simulink model "test_co_sim"  (R2020b)
settings: Solver=FixedStepDiscrete  StartTime=0.0  StopTime=10.0  FixedStep=1e-3  RelTol=1e-3
PreLoadFcn:
  | simulink_init
StopFcn:
  | % cleanup
  | if instance.reuse_instance()
  |     instance.error_shutdown("SIMULINK actor did not expect to be reused")
  | end
values from neighbouring files (symbols this model uses):
  Kd_IPF = [0 0 0 0 0 0 0 0 0 0 0 0]    [load_data.m]
  Ki_IPF = [0 0 0 0 0 0 0 0 0 0 0 0]    [load_data.m]
  Kp_IPF = [2 2 2 2 2 2 2 2 2 2 2 2]    [load_data.m]
  Maa = [0.7635    0.2320    0.0658    0.0074    0.0039    0.1363    0.0434    0.0473    0.0270    0.0150    0.0108   -0.0017 ... (first row only)    [load_data.m]
  Ra = [0         0         0         0         0         0         0         0         0         0         0         0 ... (first row only)    [load_data.m]
  T_IPF = diag([1 1 1 1 1 1 1 1 1 1 1 0].')    [load_data.m]
libraries: pid_lib x1
settings Model: Creator=ravenst1  LastModifiedBy=anandh

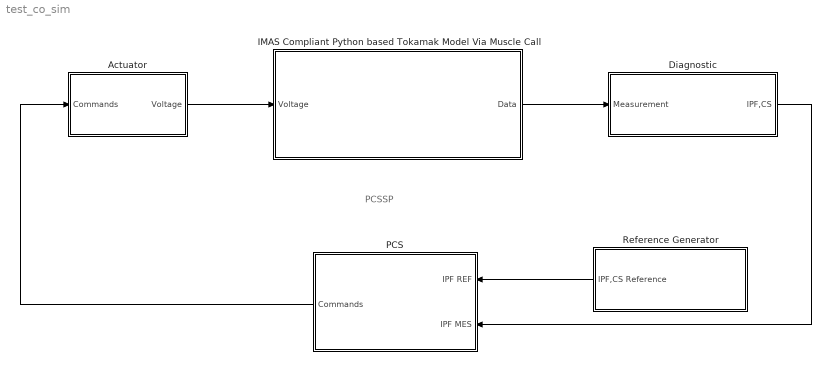
== system test_co_sim ==
  note: PCSSP
  Actuator : Subsystem
  Diagnostic : Subsystem
  "IMAS Compliant Python based Tokamak Model Via Muscle Call " : Subsystem
  PCS : Subsystem
  Reference Generator : Subsystem
  wires:
  PCS/1(Commands) -> Actuator/1(Commands)
  Actuator/1(Voltage) -> "IMAS Compliant Python based Tokamak Model Via Muscle Call "/1(Voltage)
  "IMAS Compliant Python based Tokamak Model Via Muscle Call "/1(Data) -> Diagnostic/1(Measurement)
  Diagnostic/1(IPF,CS) -> PCS/2(IPF MES)
  Reference Generator/1(IPF,CS Reference) -> PCS/1(IPF REF)

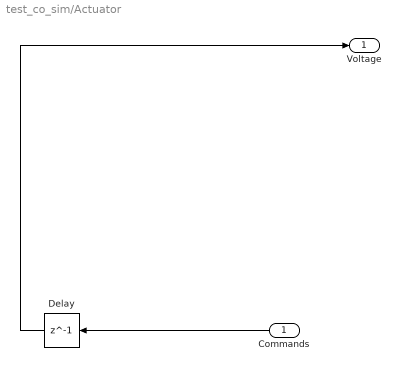
== system test_co_sim/Actuator ==
  Commands : Inport
  Delay : Delay  DelayLength=1
  Voltage : Outport
  wires:
  Commands/1 -> Delay/1
  Delay/1 -> Voltage/1

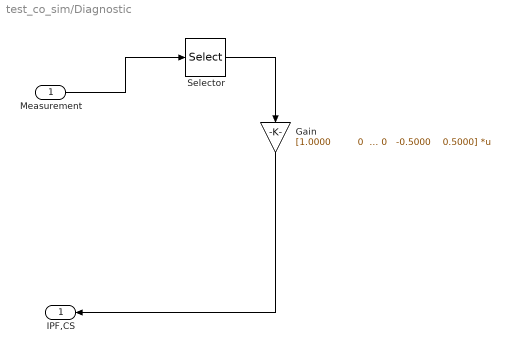
== system test_co_sim/Diagnostic ==
  Measurement : Inport
  Gain : Gain  Gain=|  Multiplication=Matrix(K*u)
      | [1.0000         0         0         0         0         0         0         0         0         0         0         0         0         0
      |          0    1.0000         0         0         0         0         0         0         0         0         0         0         0         0
      |          0         0    0.5000    0.5000         0         0         0         0         0         0         0         0         0         0
      |          0         0         0         0    1.0000         0         0         0         0         0         0         0         0         0
      |          0         0         0         0         0    1.0000         0         0         0         0         0         0         0         0
      |          0         0         0         0         0         0    1.0000         0         0         0         0         0         0         0
      |          0         0         0         0         0         0         0    1.0000         0         0         0         0         0         0
      |          0         0         0         0         0         0         0         0    1.0000         0         0         0         0         0
      |          0         0         0         0         0         0         0         0         0    1.0000         0         0         0         0
      |          0         0         0         0         0         0         0         0         0         0    1.0000         0         0         0
      |          0         0         0         0         0         0         0         0         0         0         0    1.0000         0         0
      |          0         0         0         0         0         0         0         0         0         0         0         0   -0.5000    0.5000]
  Selector : Selector  IndexOptions=Index vector (dialog)  Indices=[iter_system.output_map.cc.start:iter_system.output_map.cc.end]  OutputSizes=1
  IPF,CS : Outport
  wires:
  Selector/1 -> Gain/1
  Measurement/1 -> Selector/1
  Gain/1 -> IPF,CS/1

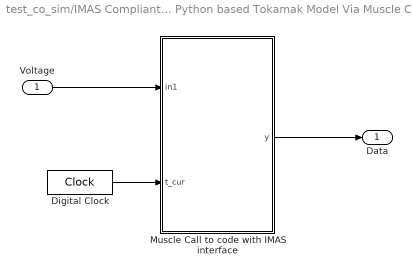
== system test_co_sim/IMAS Compliant Python based Tokamak Model Via Muscle Call  ==
  Voltage : Inport
  Digital Clock : DigitalClock  SampleTime=1e-3
  Muscle Call to code with IMAS interface : MATLAB Function  TreatAsAtomicUnit=on
  Data : Outport
  wires:
  Digital Clock/1 -> Muscle Call to code with IMAS interface/2(t_cur)
  Voltage/1 -> Muscle Call to code with IMAS interface/1(in1)
  Muscle Call to code with IMAS interface/1(y) -> Data/1

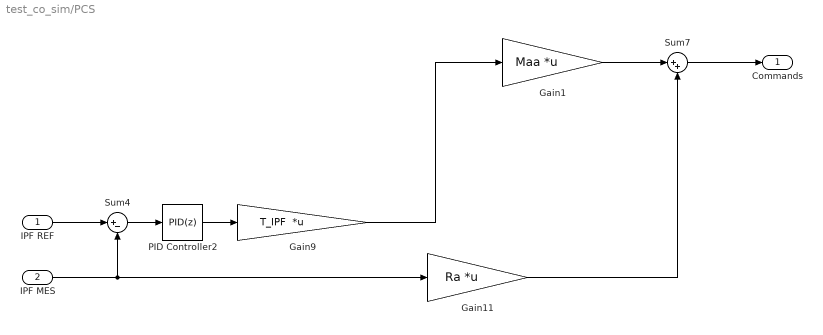
== system test_co_sim/PCS ==
  IPF REF : Inport
  IPF MES : Inport  Port=2
  Gain1 : Gain  Gain=Maa  Multiplication=Matrix(K*u)
  Gain11 : Gain  Gain=Ra  Multiplication=Matrix(K*u)
  Gain9 : Gain  Gain=T_IPF  Multiplication=Matrix(K*u)
  PID Controller2 : pid_lib/PID Controller  Controller=PID  Form=Parallel  TimeDomain=Discrete-time  UseExternalTs=off  SampleTime=-1  IntegratorMethod=Forward Euler  FilterMethod=Forward Euler  ControllerParametersSource=internal  P=Kp_IPF  I=Ki_IPF  D=Kd_IPF  UseFilter=on  N=100  TunerSelectOption=Transfer Function Based (PID Tuner App)  InitialConditionSource=internal  InitialConditionForIntegrator=0  InitialConditionForFilter=0  DifferentiatorICPrevScaledInput=0  ExternalReset=none  TrackingMode=off  Kt=1  LimitOutput=off  SatLimitsSource=internal  UpperSaturationLimit=inf  LowerSaturationLimit=-inf  LinearizeAsGain=on  AntiWindupMode=none  Kb=1  POutMin=[]  POutMax=[]  IOutMin=[]  IOutMax=[]  DOutMin=[]  DOutMax=[]  NOutMin=[]  NOutMax=[]  SumOutMin=[]  SumOutMax=[]  SaturationOutMin=[]  SaturationOutMax=[]  PParamMin=[]  PParamMax=[]  IParamMin=[]  IParamMax=[]  DParamMin=[]  DParamMax=[]  NParamMin=[]  NParamMax=[]  KbParamMin=[]  KbParamMax=[]  KtParamMin=[]  KtParamMax=[]  KbOutMin=[]  KbOutMax=[]  KtOutMin=[]  KtOutMax=[]  IntegratorOutMin=[]  IntegratorOutMax=[]  FilterOutMin=[]  FilterOutMax=[]  SumI1OutMin=[]  SumI1OutMax=[]  SumI2OutMin=[]  SumI2OutMax=[]  SumI3OutMin=[]  SumI3OutMax=[]  SumI4OutMin=[]  SumI4OutMax=[]  SumDOutMin=[]  SumDOutMax=[]  DifferentiatorOutMin=[]  DifferentiatorOutMax=[]  FilterDiffOutCoefMin=[]  FilterDiffOutCoefMax=[]  ReciprocalOutMin=[]  ReciprocalOutMax=[]  SumDenOutMin=[]  SumDenOutMax=[]  SumNumOutMin=[]  SumNumOutMax=[]  DivideOutMin=[]  DivideOutMax=[]  UdiffTsProdOutMin=[]  UdiffTsProdOutMax=[]  NTsProdOutMin=[]  NTsProdOutMax=[]  UintegralTsProdOutMin=[]  UintegralTsProdOutMax=[]  UngainTsProdOutMin=[]  UngainTsProdOutMax=[]  IntegratorContinuousStateAttributes=''  IntegratorStateMustResolveToSignalObject=off  IntegratorRTWStateStorageClass=Auto  FilterContinuousStateAttributes=''  FilterStateMustResolveToSignalObject=off  FilterRTWStateStorageClass=Auto  ParallelPVariant=InternalParameters  IdealPVariant=Disabled  IVariant=InternalParameters  DVariant=InternalParameters  IntegratorVariant=Discrete  SatVariant=Disabled  AWVariant=Passthrough  PCopyVariant=Disabled  TRVariant=Disabled  FdbkBlocksVariant=Forward  IdealPFdbkVariant=Disabled  SatFdbkVariant=Disabled  DerivativeFilterVariant=ForwardEulerFilter  NVariant=InternalParameters  NCopyVariant=Disabled  FilterICVariant=InternalICsFilter  IntegratorICVariant=InternalICs  ExternalResetVariant=Disabled  TRSumVariant=Passthrough  SumFdbkVariant=Disabled  SumVariant=Sum_PID  TsampFilterVariant=InternalTs  TsampNgainVariant=Passthrough  TsampIntegralVariant=Passthrough  ExternalSaturationOutDataTypeStr=Inherit: Same as second input
  Sum4 : Sum  Inputs=|+-
  Sum7 : Sum  Inputs=|++
  Commands : Outport
  wires:
  Sum4/1 -> PID Controller2/1
  IPF REF/1 -> Sum4/1
  Gain9/1 -> Gain1/1
  Gain11/1 -> Sum7/2
  Gain1/1 -> Sum7/1
  Sum7/1 -> Commands/1
  IPF MES/1 -> Gain11/1, Sum4/2
  PID Controller2/1 -> Gain9/1

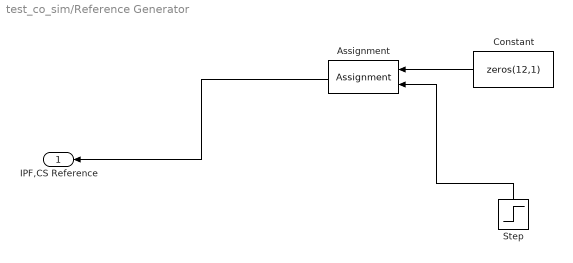
== system test_co_sim/Reference Generator ==
  Assignment : Assignment  DiagnosticForDimensions=Warning  IndexOptions=Index vector (dialog)  Indices=3  OutputSizes=1
  Constant : Constant  Value=zeros(12,1)
  Step : Step  After=1e3  SampleTime=0
  IPF,CS Reference : Outport
  wires:
  Constant/1 -> Assignment/1
  Step/1 -> Assignment/2
  Assignment/1 -> IPF,CS Reference/1

== matlab function test_co_sim/IMAS Compliant Python based Tokamak Model Via Muscle Call /Muscle Call to code with IMAS interface ==
  data: in1 input; y output; t_cur input
function y   = muscle_call(in1,t_cur)

% pre-assign output to prevent Simulink error
y = zeros(1377,1);

% constrain python function to run extrinsically in Matlab (no codegen)
coder.extrinsic('muscle_matlab_exchange');

[y] = muscle_matlab_exchange(in1,t_cur);



end
